simulink model "minimum_snap_trajectory"  (R2023b)
settings: Solver=VariableStepAuto  StartTime=0.0  StopTime=15  RelTol=1e-3
libraries: shareduavrstlib x1
settings Model: Creator=krist  LastModifiedBy=krist

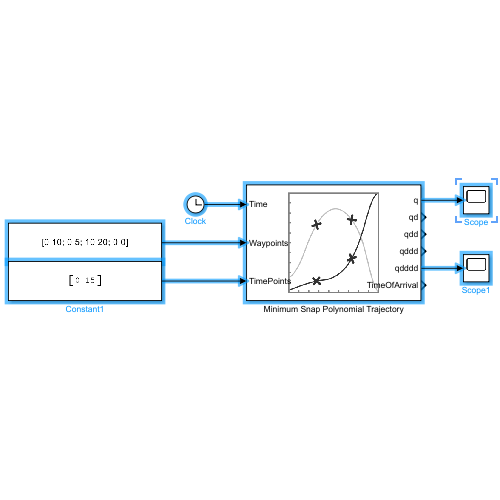
[thumbnail: Simulink's stored preview of the top-level diagram]
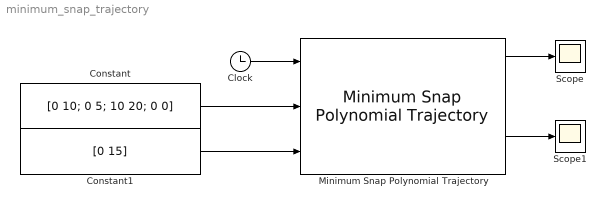
== system minimum_snap_trajectory ==
  Clock : Clock
  Constant : Constant  Value=[0 10; 0 5; 10 20; 0 0]
  Constant1 : Constant  Value=[0 15]
  Minimum Snap Polynomial Trajectory : shareduavrstlib/Minimum Snap Polynomial Trajectory  ShowBCInputPort=off  ShowPolynomialCoefs=off  ShowStatusOutputPort=off  TimeAllocation=off  TimeWeight=100  MinSegmentTime=0.1  MaxSegmentTime=1  MaxIteration=1500  MaxTime=10  SimulateUsing=Interpreted execution
      settings: LibrarySourceBlock=uavalgslib/Minimum Snap Polynomial Trajectory
  Scope : Scope
  Scope1 : Scope
  wires:
  Clock/1 -> Minimum Snap Polynomial Trajectory/1
  Constant1/1 -> Minimum Snap Polynomial Trajectory/3
  Constant/1 -> Minimum Snap Polynomial Trajectory/2
  Minimum Snap Polynomial Trajectory/1 -> Scope/1
  Minimum Snap Polynomial Trajectory/5 -> Scope1/1
